simulink model "ObtenirT3estimer"  (R2024b)
settings: Solver=VariableStepAuto  StartTime=0.0  StopTime=10.0  RelTol=1e-3
values from neighbouring files (symbols this model uses):
  f = 0.2    [matlab.mat]
undefined symbols (not defined in the file or in its folder): Z_T3
libraries: simulink_extras x1
settings Model: Creator=valun  LastModifiedBy=valun

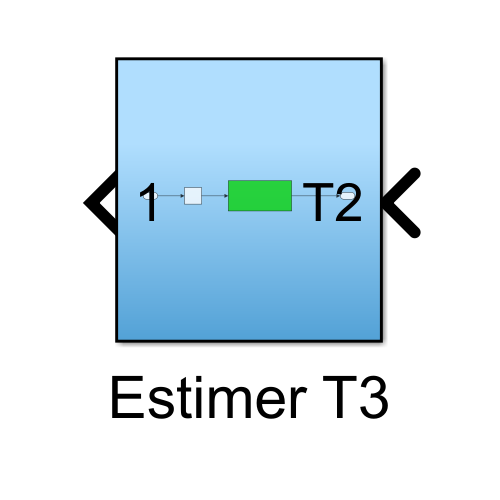
[thumbnail: Simulink's stored preview of the top-level diagram]
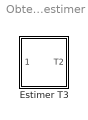
== system ObtenirT3estimer ==
  Estimer T3 : Subsystem

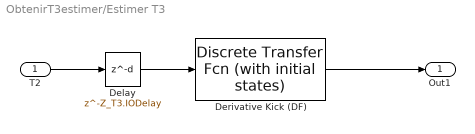
== system ObtenirT3estimer/Estimer T3 ==
  T2 : Inport
  Delay : Delay  DelayLength=Z_T3.IODelay  InitialCondition=0
  Derivative Kick (DF) : simulink_extras/Additional Discrete/Discrete Transfer Fcn (with initial states)  N=Z_T3.num{1}  D=Z_T3.den{1}  X0=[0]  TS=1/f
  Out1 : Outport
  wires:
  T2/1 -> Delay/1
  Delay/1 -> Derivative Kick (DF)/1
  Derivative Kick (DF)/1 -> Out1/1
